simulink model "Problem_3"  (R2020a)
settings: Solver=ode45  StartTime=0.0  StopTime=120  RelTol=1e-3
values from neighbouring files (symbols this model uses):
  b = 50    [Problem_3.m]    (also in Problem_3.sldd = 50.0)
  Kd = 1.0    [Problem_3.sldd]
  Ki = 170.0    [Problem_3.sldd]
  Kp = 2300.0    [Problem_3.sldd]
  m = 1000    [Problem_3.m]    (also in Problem_3.sldd = 1000.0)
settings Model: Creator=Saqlain  LastModifiedBy=Saqlain

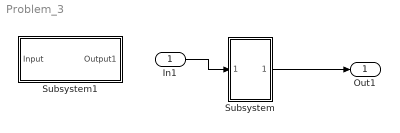
== system Problem_3 ==
  In1 : Inport
  Subsystem : Subsystem
  Subsystem1 : Subsystem
  Out1 : Outport
  wires:
  In1/1 -> Subsystem/1(In1)
  Subsystem/1(Out1) -> Out1/1

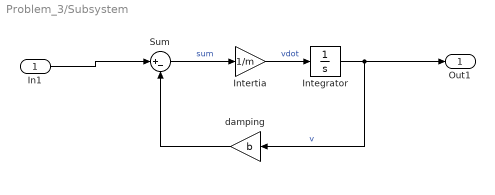
== system Problem_3/Subsystem ==
  In1 : Inport
  Integrator : Integrator
  Intertia : Gain  Gain=1/m
  Sum : Sum  Inputs=|+-
  damping : Gain  Gain=b
  Out1 : Outport
  wires:
  Sum/1 -> Intertia/1  "sum"
  Intertia/1 -> Integrator/1  "vdot"
  damping/1 -> Sum/2
  Integrator/1 -> Out1/1, damping/1  "v"
  In1/1 -> Sum/1

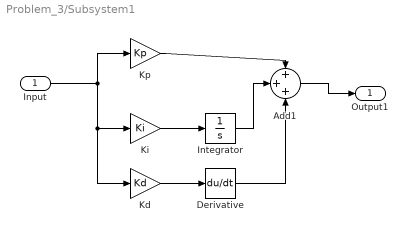
== system Problem_3/Subsystem1 ==
  Input : Inport
  Add1 : Sum  Inputs=+++
  Derivative : Derivative
  Integrator : Integrator
  Kd : Gain  Gain=Kd
  Ki : Gain  Gain=Ki
  Kp : Gain  Gain=Kp
  Output1 : Outport  OutDataTypeStr=double  PortDimensions=1  SampleTime=0
  wires:
  Integrator/1 -> Add1/2
  Kp/1 -> Add1/1
  Ki/1 -> Integrator/1
  Input/1 -> Kd/1, Ki/1, Kp/1
  Add1/1 -> Output1/1
  Derivative/1 -> Add1/3
  Kd/1 -> Derivative/1
